simulink model "IMUsimss"  (R2025b)
settings: Solver=VariableStepAuto  StartTime=0.0  StopTime=10.0  FixedStep=0.01  RelTol=1e-3
settings Model: Creator=2005B  LastModifiedBy=2005B

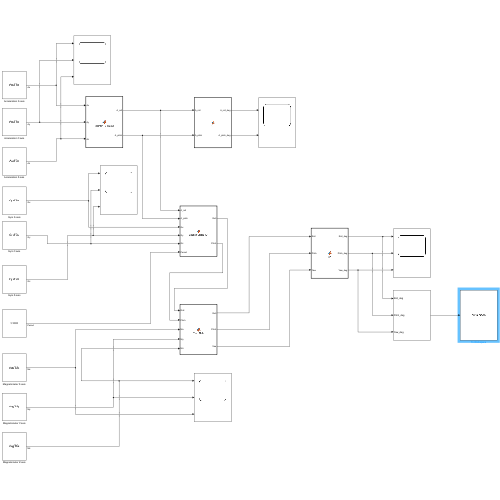
[thumbnail: Simulink's stored preview of the top-level diagram]
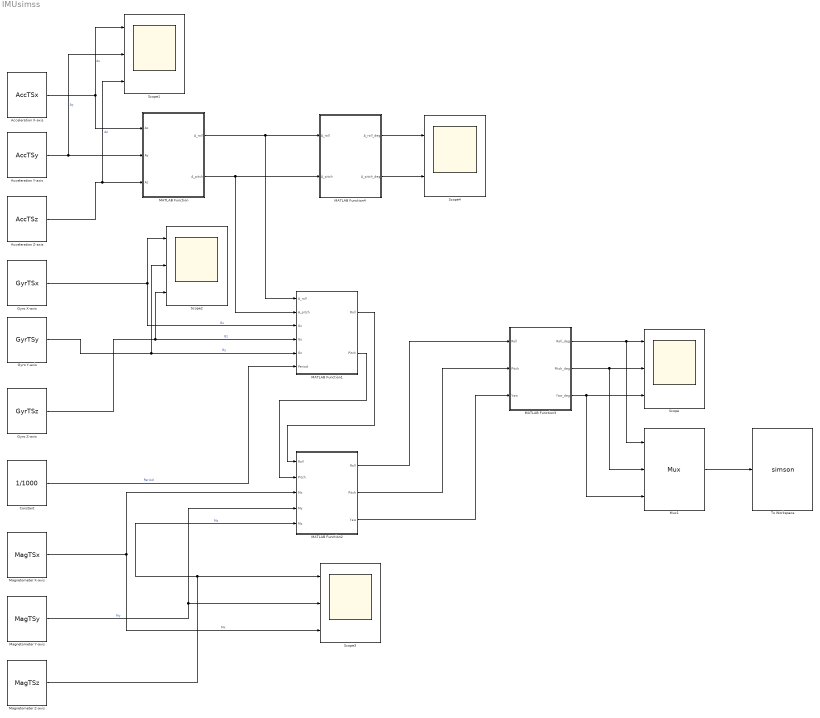
== system IMUsimss ==
  Acceleration X-axis : FromWorkspace  VariableName=AccTSx  SampleTime=0.001  OutputAfterFinalValue=Holding final value
  Acceleration Y-axis : FromWorkspace  VariableName=AccTSy  SampleTime=0.001  OutputAfterFinalValue=Holding final value
  Acceleration Z-axis : FromWorkspace  VariableName=AccTSz  SampleTime=0.001  OutputAfterFinalValue=Holding final value
  Constant : Constant  Value=1/1000
  Gyro X-axis : FromWorkspace  VariableName=GyrTSx  SampleTime=0.001  OutputAfterFinalValue=Holding final value
  Gyro Y-axis : FromWorkspace  VariableName=GyrTSy  SampleTime=0.001  OutputAfterFinalValue=Holding final value
  Gyro Z-axis : FromWorkspace  VariableName=GyrTSz  SampleTime=0.001  OutputAfterFinalValue=Holding final value
  MATLAB Function : MATLAB Function  TreatAsAtomicUnit=on
  MATLAB Function1 : MATLAB Function  TreatAsAtomicUnit=on
  MATLAB Function2 : MATLAB Function  TreatAsAtomicUnit=on
  MATLAB Function3 : MATLAB Function  TreatAsAtomicUnit=on
  MATLAB Function4 : MATLAB Function  TreatAsAtomicUnit=on
  Magnetometer X-axis : FromWorkspace  VariableName=MagTSx  SampleTime=0.001  OutputAfterFinalValue=Holding final value
  Magnetometer Y-axis : FromWorkspace  VariableName=MagTSy  SampleTime=0.001  OutputAfterFinalValue=Holding final value
  Magnetometer Z-axis : FromWorkspace  VariableName=MagTSz  SampleTime=0.001  OutputAfterFinalValue=Holding final value
  Mux1 : Mux  Inputs=3
      settings: DisplayOption=signals
  Scope{,1..3} (4 alike) : Scope  NumInputPorts=3
      Scope settings: SampleTime=0.001  ActiveDisplayYMinimum=-626.07248620617906  ActiveDisplayYMaximum=849.47998762379711  DataLoggingVariableName=imu_scope
      Scope1 settings: SampleTime=0.001  ActiveDisplayYMinimum=-15.672532818277128  ActiveDisplayYMaximum=12.5511454334419  YLabel=Acceleration (m/s^2)
      Scope2 settings: SampleTime=0.001  ActiveDisplayYMinimum=-4.5175958238523037  ActiveDisplayYMaximum=8.3461729143268446  DataLoggingVariableName=ScopeData2
      Scope3 settings: SampleTime=0.001  ActiveDisplayYMinimum=-200  ActiveDisplayYMaximum=200  DataLoggingVariableName=ScopeData3
  Scope4 : Scope  NumInputPorts=2
      settings: SampleTime=0.001  ActiveDisplayYMinimum=-15  YLabel=Acceleration (m/s^2)  DataLoggingVariableName=ScopeData4
  To Workspace : ToWorkspace  VariableName=simson  SaveFormat=Structure With Time  SampleTime=0.001
  wires:
  Acceleration Y-axis/1 -> Scope1/2, MATLAB Function/2(Ay)  "Ay"
  Acceleration X-axis/1 -> Scope1/1, MATLAB Function/1(Ax)  "Ax"
  Acceleration Z-axis/1 -> Scope1/3, MATLAB Function/3(Az)  "Az"
  MATLAB Function/1(A_roll) -> MATLAB Function1/1(A_roll), MATLAB Function4/1(A_roll)
  MATLAB Function/2(A_pitch) -> MATLAB Function1/2(A_pitch), MATLAB Function4/2(A_pitch)
  Gyro X-axis/1 -> Scope2/1, MATLAB Function1/3(Gx)  "Gx"
  Gyro Y-axis/1 -> MATLAB Function1/5(Gz), Scope2/2  "Gy"
  Gyro Z-axis/1 -> Scope2/3, MATLAB Function1/4(Gy)  "Gz"
  Constant/1 -> MATLAB Function1/6(Period)  "Period"
  Magnetometer X-axis/1 -> MATLAB Function2/3(Mx), Scope3/3  "Mx"
  Magnetometer Y-axis/1 -> Scope3/2, MATLAB Function2/4(My)  "My"
  Magnetometer Z-axis/1 -> MATLAB Function2/5(Mz), Scope3/1  "Mz"
  MATLAB Function1/1(Roll) -> MATLAB Function2/1("Roll ")
  MATLAB Function1/2(Pitch) -> MATLAB Function2/2("Pitch ")
  MATLAB Function2/2(Pitch) -> MATLAB Function3/2(Pitch)
  MATLAB Function2/1(Roll) -> MATLAB Function3/1(Roll)
  MATLAB Function2/3(Yaw) -> MATLAB Function3/3(Yaw)
  MATLAB Function3/2(Pitch_deg) -> Scope/2, Mux1/2
  MATLAB Function3/3(Yaw_deg) -> Scope/3, Mux1/3
  MATLAB Function3/1(Roll_deg) -> Scope/1, Mux1/1
  MATLAB Function4/2(A_pitch_deg) -> Scope4/2
  MATLAB Function4/1(A_roll_deg) -> Scope4/1
  Mux1/1 -> To Workspace/1

== matlab function IMUsimss/MATLAB Function1 ==
  data: A_roll input; Roll output; A_pitch input; Gx input; Gy input; Gz input; Period input; Pitch output
function [Roll, Pitch] = SensorFusion_KF(A_roll, A_pitch, Gx, Gy, Gz, Period)

% State: x = [phi; theta; psi]
persistent H Q R x_hat P inited
if isempty(inited)
    H = [1 0 0;   % measure phi
         0 1 0];  % measure theta

    Q = diag([1e-4, 1e-4, 1e-1]);   % process noise (tune)
    R = 10.0 * eye(2);              % meas noise (tune)

    x_hat = [0;0;0];                % [phi; theta; psi] (rad)
    P     = 10.0 * eye(3);
    inited = true;
end

% Inputs
z = [A_roll; A_pitch];    % <-- column vector (2x1)
p = Gx; q = Gy; r = Gz;
dt = Period;

% ---- Predict
A = Ajacob(x_hat, p, q, r, dt);
xp = fx(x_hat, p, q, r, dt);
Pp = A*P*A' + Q;

% ---- Update
S = H*Pp*H' + R;          % innovation covariance (2x2)
K = (Pp*H') / S;          % numerically stable (instead of inv)

innov = z - H*xp;         % (2x1)
x_hat = xp + K*innov;     % (3x1)

I = eye(3);               % Joseph-form covariance update
P = (I - K*H)*Pp*(I - K*H)' + K*R*K';

% Outputs
Roll  = x_hat(1);
Pitch = x_hat(2);

% --------- Local functions ---------
function xp = fx(xhat, p, q, r, dt)
phi = xhat(1); theta = xhat(2);
% guard against cos(theta) -> 0
ct = cos(theta); if abs(ct) < 1e-6, ct = sign(ct)*1e-6; end
xdot = zeros(3,1);
xdot(1) = p + q*sin(phi)*tan(theta) + r*cos(phi)*tan(theta);
xdot(2) = q*cos(phi) - r*sin(phi);
xdot(3) = q*sin(phi)/ct + r*cos(phi)/ct;
xp = xhat + xdot*dt;

function A = Ajacob(xhat, p, q, r, dt)
phi = xhat(1); theta = xhat(2);
ct = cos(theta); st = sin(theta);
% avoid division blow-up
if abs(ct) < 1e-6, ct = sign(ct)*1e-6; end
sec2 = 1/(ct*ct);
A = zeros(3,3);
A(1,1) = q*cos(phi)*tan(theta) - r*sin(phi)*tan(theta);
A(1,2) = (q*sin(phi) + r*cos(phi))*sec2;
A(2,1) = -q*sin(phi) - r*cos(phi);
A(3,1) = q*cos(phi)/ct - r*sin(phi)/ct;
A(3,2) = (q*sin(phi) + r*cos(phi))*sec2*tan(theta);
A = eye(3) + A*dt;

== matlab function IMUsimss/MATLAB Function ==
  data: Ax input; Ay input; Az input; A_roll output; A_pitch output
function [A_roll, A_pitch] = RollPitch_Baseline(Ax, Ay, Az)

A_roll = atan2(Ay, Az);
A_pitch = atan2(-Ax,sqrt((Ay*Ay) + (Az*Az)));

== matlab function IMUsimss/MATLAB Function2 ==
  data: Roll input; Pitch input; Mx input; My input; Mz input; Roll output; Pitch output; Yaw output
function [Roll, Pitch, Yaw] = Yaw_Calc(Roll, Pitch, Mx, My, Mz)

    By = Mz*sin(Roll) - My*cos(Roll);
    Bx = Mx*cos(Pitch) + My*sin(Pitch)*sin(Roll) + Mz*sin(Pitch)*cos(Roll);

    Yaw = atan2(-By, Bx);   % add declination here if you want true heading
end

== matlab function IMUsimss/MATLAB Function3 ==
  data: Roll input; Pitch input; Roll_deg output; Yaw input; Pitch_deg output; Yaw_deg output
function [Roll_deg, Pitch_deg, Yaw_deg] = fcn(Roll, Pitch, Yaw)
    Roll_deg  = rad2deg(wrapToPi(Roll));
    Pitch_deg = rad2deg(wrapToPi(Pitch));
    Yaw_deg   = rad2deg(wrapToPi(Yaw));
end

== matlab function IMUsimss/MATLAB Function4 ==
  data: A_roll input; A_roll_deg output; A_pitch input; A_pitch_deg output
function [A_roll_deg, A_pitch_deg] = fcn(A_roll, A_pitch)

A_roll_deg = A_roll * (180/pi);
A_pitch_deg = A_pitch * (180/pi);
